simulink model "Reg_courant_RL_H26_2024"  (R2024a)
settings: Solver=ode4  StartTime=0.0  StopTime=inf  FixedStep=Ts  RelTol=1e-3
PostLoadFcn:
  | Reg_vitesse_courant_H24m;
InitFcn:
  | Reg_courant_RL_H26m;
values from neighbouring files (symbols this model uses):
  fperturbation = 1 / (2*pi*nc*Tel)    (= 200.494258843)    [Reg_courant_RL_H26m.m]
  Ian = 0.5    [Reg_courant_RL_H26m.m]
  Kamp = Gain_Ampli_Puissance(1)    [Reg_courant_RL_H26m.m]
  Kc = Gain_Capteur_Courant(1)    [Reg_courant_RL_H26m.m]
  Kel = 1 / Rel    (= 0.283808712927)    [Reg_courant_RL_H26m.m]
  limVampinf = -5    [Reg_courant_RL_H26m.m]
  limVampsup = 5    [Reg_courant_RL_H26m.m]
  PulseWidth = Tperturbcourant / 2    [Reg_courant_RL_H26m.m]
  Tech = Tel / nTechTel    [Reg_courant_RL_H26m.m]
  Tel = Lel / Rel    (= 7.93812970058e-05)    [Reg_courant_RL_H26m.m]
  Tperturbcourant = 4 * ceil(Ntau * Tel / Ts)    [Reg_courant_RL_H26m.m]
  Ts = Tel / nTsTel    (= 1.98453242515e-06)    [Reg_courant_RL_H26m.m]
libraries: simulink x4, slpidlib x2
settings Model: Creator=Philippe Viarouge  LastModifiedBy=guill
settings SolverCC: AlgebraicLoopSolver=TrustRegion
settings ModelReferenceCC: EnableRefExpFcnMdlSchedulingChecks=on
settings RTWCC: GPUComputeCapability=3.5  DLArmComputeVersion=19.05
settings ConfigComp: CovBoundaryAbsTol=1.0e-5

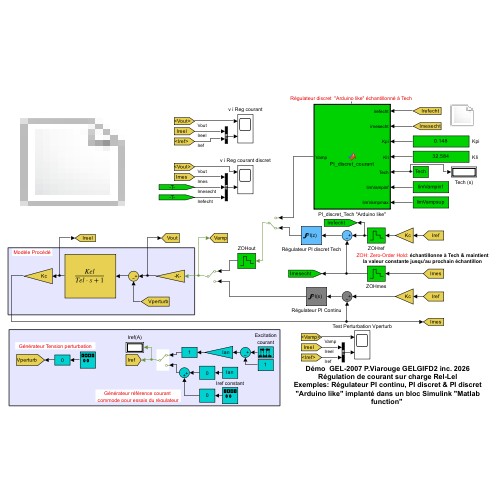
[thumbnail: Simulink's stored preview of the top-level diagram]
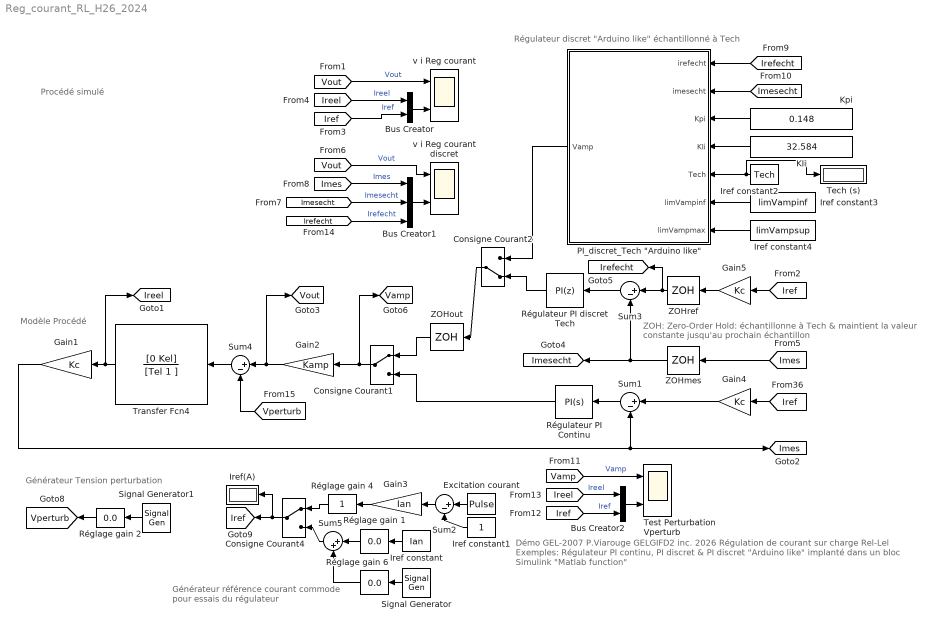
== system Reg_courant_RL_H26_2024 ==
  note: Modèle Procédé
  note: Générateur référence courant
      | commode pour essais du régulateur
  note: Générateur Tension perturbation
  note: Régulateur discret "Arduino like" échantillonné à Tech
  note: Procédé simulé
  note: Démo  GEL-2007 P.Viarouge GELGIFD2 inc. 2026
      | Régulation de courant sur charge Rel-Lel
      | Exemples: Régulateur PI continu, PI discret & PI discret "Arduino like" implanté dans un bloc Simulink "Matlab function"
  note: ZOH: Zero-Order Hold: échantillonne à Tech & maintient la valeur constante jusqu'au prochain échantillon
  " Consigne Courant1" : ManualSwitch
  " Consigne Courant2" : ManualSwitch  CurrentSetting=0
  " Consigne Courant4" : ManualSwitch
  Bus Creator : BusCreator  Inputs=2
  Bus Creator1 : BusCreator  Inputs=3
  Bus Creator2 : BusCreator  Inputs=2
  Excitation courant : DiscretePulseGenerator  Amplitude=2  Period=Tperturbcourant  PulseWidth=PulseWidth  PhaseDelay=PulseWidth  SampleTime=Ts
  Gain1 : Gain  Gain=Kc  SaturateOnIntegerOverflow=on  OutDataTypeStr=Inherit: Same as input  ParamDataTypeStr=Inherit: Same as input
  Gain2 : Gain  Gain=Kamp  SaturateOnIntegerOverflow=on  OutDataTypeStr=Inherit: Same as input  ParamDataTypeStr=Inherit: Same as input
  Gain3 : Gain  Gain=Ian  SaturateOnIntegerOverflow=on  OutDataTypeStr=Inherit: Same as input  ParamDataTypeStr=Inherit: Same as input
  Gain4 : Gain  Gain=Kc  SaturateOnIntegerOverflow=on  OutDataTypeStr=Inherit: Same as input  ParamDataTypeStr=Inherit: Same as input
  Gain5 : Gain  Gain=Kc  SaturateOnIntegerOverflow=on  OutDataTypeStr=Inherit: Same as input  ParamDataTypeStr=Inherit: Same as input
  Iref constant : Constant  Value=Ian
  Iref constant1 : Constant
  Iref constant2 : Constant  Value=Tech
  Iref constant3 : Constant  Value=limVampinf
  Iref constant4 : Constant  Value=limVampsup
  Iref(A) : Display
  KIi : Constant  Value=32.584
  Kpi : Constant  Value=0.148
  "PI_discret_Tech \"Arduino like\"" : MATLAB Function  TreatAsAtomicUnit=on
  Réglage gain 1 : simulink/Math Operations/Slider Gain  gain=0.0  low=0  high=1
  Réglage gain 2 : simulink/Math Operations/Slider Gain  gain=0.0  low=0  high=10
  Réglage gain 4 : simulink/Math Operations/Slider Gain  gain=1  low=0  high=2
  Réglage gain 6 : simulink/Math Operations/Slider Gain  gain=0.0  low=0  high=2
  Régulateur PI Continu : slpidlib/PID Controller  Controller=PI  Form=Parallel  TimeDomain=Continuous-time  UseExternalTs=off  SampleTime=Ts  IntegratorMethod=Forward Euler  FilterMethod=Forward Euler  ControllerParametersSource=internal  P=2.13202399414714  I=58536.4727696562  UseKiTs=off  D=-0.000553625934463325  UseExternalDerivativeSource=off  N=711.832973902977  UseFilter=on  TunerSelectOption=Transfer Function Based (PID Tuner App)  InitialConditionSource=internal  InitialConditionForIntegrator=0  InitialConditionForFilter=0  DifferentiatorICPrevScaledInput=0  ExternalReset=none  TrackingMode=off  Kt=1  LimitOutput=on  SatLimitsSource=internal  UpperSaturationLimit=limVampsup  LowerSaturationLimit=limVampinf  LinearizeAsGain=off  AntiWindupMode=clamping  Kb=1  LimitIntegrator=off  UpperIntegratorSaturationLimit=inf  LowerIntegratorSaturationLimit=-inf  POutMin=[]  POutMax=[]  IOutMin=[]  IOutMax=[]  DOutMin=[]  DOutMax=[]  NOutMin=[]  NOutMax=[]  SumOutMin=[]  SumOutMax=[]  SaturationOutDataTypeStr=Inherit: Inherit via back propagation  SaturationOutMin=[]  SaturationOutMax=[]  PParamMin=[]  PParamMax=[]  IParamMin=[]  IParamMax=[]  DParamMin=[]  DParamMax=[]  NParamMin=[]  NParamMax=[]  KbParamMin=[]  KbParamMax=[]  KtParamMin=[]  KtParamMax=[]  KbOutMin=[]  KbOutMax=[]  KtOutMin=[]  KtOutMax=[]  IntegratorOutMin=[]  IntegratorOutMax=[]  FilterOutMin=[]  FilterOutMax=[]  SumI1OutMin=[]  SumI1OutMax=[]  SumI2OutMin=[]  SumI2OutMax=[]  SumI3OutMin=[]  SumI3OutMax=[]  SumI4OutMin=[]  SumI4OutMax=[]  SumDOutMin=[]  SumDOutMax=[]  DifferentiatorOutMin=[]  DifferentiatorOutMax=[]  FilterDiffOutCoefMin=[]  FilterDiffOutCoefMax=[]  ReciprocalOutMin=[]  ReciprocalOutMax=[]  SumDenOutMin=[]  SumDenOutMax=[]  SumNumOutMin=[]  SumNumOutMax=[]  DivideOutMin=[]  DivideOutMax=[]  UdiffTsProdOutMin=[]  UdiffTsProdOutMax=[]  NTsProdOutMin=[]  NTsProdOutMax=[]  UintegralTsProdOutMin=[]  UintegralTsProdOutMax=[]  UngainTsProdOutMin=[]  UngainTsProdOutMax=[]  ClampingZeroOutDataTypeStr=Inherit: Inherit via back propagation  ClampingZeroOutMin=[]  ClampingZeroOutMax=[]  FilterDenConstantOutDataTypeStr=Inherit: Inherit via back propagation  FilterDenConstantOutMin=[]  FilterDenConstantOutMax=[]  PCopyOutDataTypeStr=Inherit: Inherit via back propagation  PCopyOutMin=[]  PCopyOutMax=[]  NCopyOutDataTypeStr=Inherit: Inherit via back propagation  NCopyOutMin=[]  NCopyOutMax=[]  IntegratorContinuousStateAttributes=''  IntegratorStateMustResolveToSignalObject=off  IntegratorRTWStateStorageClass=Auto  FilterContinuousStateAttributes=''  FilterStateMustResolveToSignalObject=off  FilterRTWStateStorageClass=Auto  ParallelPVariant=InternalParameters  IdealPVariant=Disabled  IVariant=InternalParameters  DVariant=Disabled  IntegratorVariant=Continuous  SatVariant=Enabled  AWVariant=ContClampingParallel  PCopyVariant=Disabled  TRVariant=Disabled  FdbkBlocksVariant=Forward  IdealPFdbkVariant=Disabled  SatFdbkVariant=Disabled  DerivativeFilterVariant=Disabled  NVariant=Disabled  NCopyVariant=Disabled_SignalSpec  FilterICVariant=Disabled  IntegratorICVariant=InternalICs  ExternalResetVariant=Disabled  TRSumVariant=Passthrough  SumFdbkVariant=Disabled  SumVariant=Sum_PI  TsampFilterVariant=InternalTs  TsampNgainVariant=Passthrough  TsampIntegralVariant=Disabled_SignalSpec  ExternalSaturationOutDataTypeStr=Inherit: Same as second input  DerivativeSourceVariant=Disabled
  Régulateur PI discret Tech : slpidlib/PID Controller  Controller=PI  Form=Parallel  TimeDomain=Discrete-time  UseExternalTs=off  SampleTime=Tech  IntegratorMethod=Forward Euler  FilterMethod=Forward Euler  ControllerParametersSource=internal  P=2.13202399414714  I=58536.4727696562  UseKiTs=off  D=-0.000553625934463325  UseExternalDerivativeSource=off  N=711.832973902977  UseFilter=on  TunerSelectOption=Transfer Function Based (PID Tuner App)  InitialConditionSource=internal  InitialConditionForIntegrator=0  InitialConditionForFilter=0  DifferentiatorICPrevScaledInput=0  ExternalReset=none  TrackingMode=off  Kt=1  LimitOutput=on  SatLimitsSource=internal  UpperSaturationLimit=limVampsup  LowerSaturationLimit=limVampinf  LinearizeAsGain=off  AntiWindupMode=clamping  Kb=1  LimitIntegrator=off  UpperIntegratorSaturationLimit=inf  LowerIntegratorSaturationLimit=-inf  POutMin=[]  POutMax=[]  IOutMin=[]  IOutMax=[]  DOutMin=[]  DOutMax=[]  NOutMin=[]  NOutMax=[]  SumOutMin=[]  SumOutMax=[]  SaturationOutDataTypeStr=Inherit: Inherit via back propagation  SaturationOutMin=[]  SaturationOutMax=[]  PParamMin=[]  PParamMax=[]  IParamMin=[]  IParamMax=[]  DParamMin=[]  DParamMax=[]  NParamMin=[]  NParamMax=[]  KbParamMin=[]  KbParamMax=[]  KtParamMin=[]  KtParamMax=[]  KbOutMin=[]  KbOutMax=[]  KtOutMin=[]  KtOutMax=[]  IntegratorOutMin=[]  IntegratorOutMax=[]  FilterOutMin=[]  FilterOutMax=[]  SumI1OutMin=[]  SumI1OutMax=[]  SumI2OutMin=[]  SumI2OutMax=[]  SumI3OutMin=[]  SumI3OutMax=[]  SumI4OutMin=[]  SumI4OutMax=[]  SumDOutMin=[]  SumDOutMax=[]  DifferentiatorOutMin=[]  DifferentiatorOutMax=[]  FilterDiffOutCoefMin=[]  FilterDiffOutCoefMax=[]  ReciprocalOutMin=[]  ReciprocalOutMax=[]  SumDenOutMin=[]  SumDenOutMax=[]  SumNumOutMin=[]  SumNumOutMax=[]  DivideOutMin=[]  DivideOutMax=[]  UdiffTsProdOutMin=[]  UdiffTsProdOutMax=[]  NTsProdOutMin=[]  NTsProdOutMax=[]  UintegralTsProdOutMin=[]  UintegralTsProdOutMax=[]  UngainTsProdOutMin=[]  UngainTsProdOutMax=[]  ClampingZeroOutDataTypeStr=Inherit: Inherit via back propagation  ClampingZeroOutMin=[]  ClampingZeroOutMax=[]  FilterDenConstantOutDataTypeStr=Inherit: Inherit via back propagation  FilterDenConstantOutMin=[]  FilterDenConstantOutMax=[]  PCopyOutDataTypeStr=Inherit: Inherit via back propagation  PCopyOutMin=[]  PCopyOutMax=[]  NCopyOutDataTypeStr=Inherit: Inherit via back propagation  NCopyOutMin=[]  NCopyOutMax=[]  IntegratorContinuousStateAttributes=''  IntegratorStateMustResolveToSignalObject=off  IntegratorRTWStateStorageClass=Auto  FilterContinuousStateAttributes=''  FilterStateMustResolveToSignalObject=off  FilterRTWStateStorageClass=Auto  ParallelPVariant=InternalParameters  IdealPVariant=Disabled  IVariant=InternalParameters  DVariant=Disabled  IntegratorVariant=Discrete  SatVariant=Enabled  AWVariant=DiscClampingParallel  PCopyVariant=Disabled  TRVariant=Disabled  FdbkBlocksVariant=Forward  IdealPFdbkVariant=Disabled  SatFdbkVariant=Disabled  DerivativeFilterVariant=Disabled  NVariant=Disabled  NCopyVariant=Disabled_SignalSpec  FilterICVariant=Disabled  IntegratorICVariant=InternalICs  ExternalResetVariant=Disabled  TRSumVariant=Passthrough  SumFdbkVariant=Disabled  SumVariant=Sum_PI  TsampFilterVariant=InternalTs  TsampNgainVariant=Passthrough  TsampIntegralVariant=Disabled_SignalSpec  ExternalSaturationOutDataTypeStr=Inherit: Same as second input  DerivativeSourceVariant=Disabled
  Signal Generator : SignalGenerator  Amplitude=Ian  Frequency=10
  Signal Generator1 : SignalGenerator  Frequency=fperturbation
  Sum{1..4} (4 alike) : Sum  Inputs=|+-
  Sum5 : Sum  Inputs=|++
  Tech (s) : Display
  Test Perturbation Vperturb : Scope  NumInputPorts=2
  Transfer Fcn4 : TransferFcn  Numerator=[0 Kel]  Denominator=[Tel 1 ]
  ZOHmes : ZeroOrderHold  SampleTime=Tech
  ZOHout : ZeroOrderHold  SampleTime=Tech
  ZOHref : ZeroOrderHold  SampleTime=Tech
  v i Reg courant : Scope  NumInputPorts=2
  v i Reg courant discret : Scope  NumInputPorts=2
  tag scope: Imes=global, Imesecht=global, Ireel=global, Iref=global, Irefecht=global, Vamp=global, Vout=global, Vperturb=global
  wires:
  Réglage gain 1/1 -> Sum5/1
  Sum5/1 -> " Consigne Courant4"/2
  Iref constant/1 -> Réglage gain 1/1
  Gain1/1 -> Sum1/2, [Imes]
  Réglage gain 4/1 -> " Consigne Courant4"/1
  Gain3/1 -> Réglage gain 4/1
  Gain4/1 -> Sum1/1
  Signal Generator/1 -> Réglage gain 6/1
  Transfer Fcn4/1 -> [Ireel], Gain1/1
  Réglage gain 6/1 -> Sum5/2
  [Iref] -> Gain4/1
  [Vout] -> v i Reg courant/1  "Vout"
  [Ireel] -> Bus Creator/1  "Ireel"
  [Iref] -> Bus Creator/2  "Iref"
  Bus Creator/1 -> v i Reg courant/2
  Excitation courant/1 -> Sum2/1
  Iref constant1/1 -> Sum2/2
  Sum2/1 -> Gain3/1
  Sum1/1 -> Régulateur PI Continu/1
  Régulateur PI Continu/1 -> " Consigne Courant1"/2
  Sum3/1 -> Régulateur PI discret Tech/1
  ZOHref/1 -> [Irefecht], Sum3/1
  ZOHmes/1 -> Sum3/2, [Imesecht]
  [Imes] -> ZOHmes/1
  ZOHout/1 -> " Consigne Courant1"/1
  Gain5/1 -> ZOHref/1
  [Iref] -> Gain5/1
  Bus Creator1/1 -> v i Reg courant discret/2
  [Imesecht] -> Bus Creator1/2  "Imesecht"
  [Vout] -> v i Reg courant discret/1  "Vout"
  [Imes] -> Bus Creator1/1  "Imes"
  [Irefecht] -> "PI_discret_Tech \"Arduino like\""/1(irefecht)
  [Imesecht] -> "PI_discret_Tech \"Arduino like\""/2(imesecht)
  "PI_discret_Tech \"Arduino like\""/1(Vamp) -> " Consigne Courant2"/1
  " Consigne Courant2"/1 -> ZOHout/1
  Régulateur PI discret Tech/1 -> " Consigne Courant2"/2
  Kpi/1 -> "PI_discret_Tech \"Arduino like\""/3(Kpi)
  KIi/1 -> "PI_discret_Tech \"Arduino like\""/4(KIi)
  Iref constant2/1 -> "PI_discret_Tech \"Arduino like\""/5(Tech), Tech (s)/1
  Iref constant3/1 -> "PI_discret_Tech \"Arduino like\""/6(limVampinf)
  Iref constant4/1 -> "PI_discret_Tech \"Arduino like\""/7(limVampmax)
  Sum4/1 -> Transfer Fcn4/1
  Gain2/1 -> [Vout], Sum4/1
  " Consigne Courant1"/1 -> Gain2/1, [Vamp]
  [Vamp] -> Test Perturbation Vperturb/1  "Vamp"
  Bus Creator2/1 -> Test Perturbation Vperturb/2
  [Iref] -> Bus Creator2/2  "Iref"
  [Ireel] -> Bus Creator2/1  "Ireel"
  [Irefecht] -> Bus Creator1/3  "Irefecht"
  Signal Generator1/1 -> Réglage gain 2/1
  Réglage gain 2/1 -> [Vperturb]
  [Vperturb] -> Sum4/2
  " Consigne Courant4"/1 -> Iref(A)/1, [Iref]

== matlab function Reg_courant_RL_H26_2024/PI_discret_Tech "Arduino like" ==
  data: irefecht input; Vamp output; imesecht input; Kpi input; KIi input; Tech input; limVampinf input; limVampmax input
function Vamp = PI_discret_courant(irefecht, imesecht, Kpi, KIi, Tech, limVampinf, limVampmax)
%P.Viarouge 06-03-26
% Régulateur PI discret à intégrateur explicite pour régulation de courant
%
% Remarque : les paramètres du régulateur (gains Kpi, KIi, période
% d'échantillonnage Tech, seuils des limiteurs de sortie du régulateur
% limVampinf et limVampmax) sont déclarés comme arguments de la fonction.
% Dans le bloc MATLAB Function de Simulink, ils apparaissent donc comme
% des entrées du bloc.
%
% Cela permet de relier ces entrées à des blocs Constant de Simulink,
% ce qui rend le réglage du régulateur simple et visible directement
% dans le schéma.
%
% Cette méthode est souvent plus pratique que de déclarer ces paramètres
% comme des variables internes ou des paramètres du bloc dans l’éditeur
% de la MATLAB Function, car elle permet d’ajuster les gains du régulateur
% directement depuis le modèle Simulink en changeant les valeurs de ces
% variables dans les blocs Constant "à la volée" pendant la simulation
% en mode permanent (avec StopTime = tinf).
%
% ENTREES :
%   irefecht   : courant de référence échantillonné (ZOH à Tech)
%   imesecht   : courant mesuré échantillonné (ZOH à Tech)
%   Kpi        : gain proportionnel du PI
%   KIi        : gain intégral du PI
%   Tech       : période d'échantillonnage
%   limVampinf : limite basse de la commande : limiteur de sortie du PI
%   limVampmax : limite haute de la commande : limiteur de sortie du PI
%
% SORTIE :
%   Vamp       : signal de commande amplificateur de gain Kamp
%
% EQUATIONS DISCRETES DU PI IMPLANTEES :
%   e(k)        = irefecht(k) - imesecht(k)     % erreur de courant
%   xI(k)       = xI(k-1) + Tech*e(k)           % état intégrateur discret
%   Vamp_ns(k)  = Kpi*e(k) + KIi*xI(k)          % commande non saturée
%   Vamp(k)     = saturation( Vamp_ns(k) )      % commande réellement appliquée
%
% Ici, l'intégrateur est explicite : la variable xI représente directement
% l'intégrale discrète de l'erreur. Cela rend l'interprétation physique
% et la gestion de l'anti-windup plus claires
%
% Variables persistantes = mémoire du régulateur entre deux échantillons
% prélevés à Tech. Variables déclarées persistent dans la fonction.
% Signification : elles conservent leur valeur entre deux appels
% de la fonction.
%
% xIi    : état intégrateur discret du régulateur
% eiprec : erreur précédente (utile ici surtout pour mémoire/observation,
%          même si la formulation PI explicite de l'intégrateur 
%          n'en a pas nécessairement besoin)
persistent xIi eiprec

% Initialisation xIi et eiprec au début de la simulation
% Au premier appel de la fonction, ces variables persistent n’existent pas
% encore. Elles sont donc vides. La fonction isempty() permet de détecter
% cette situation.
if isempty(xIi)
    xIi = 0;
end
if isempty(eiprec)
    eiprec = 0;
end

% Calcul de l'erreur de courant pour l'échantillon courant
ei = irefecht - imesecht;

% -------------------------------------------------------------------------
% CALCUL PROVISOIRE DE L'ETAT INTEGRATEUR
% On calcule d'abord la valeur "candidate" de l'intégrateur à l'instant k :
% xIi_new = xIi(k-1) + Tech*e(k)
%
% Cette valeur n'est pas encore validée définitivement car on doit d'abord
% vérifier si elle conduit à une commande non saturée qui aggrave
% une saturation déjà présente.
% -------------------------------------------------------------------------
xIi_new = xIi + Tech*ei;

% Calcul de la commande "non saturée" (la saturation est appliquée après)
% Vamp_ns : commande calculée par le PI avant limitation
Vamp_ns = Kpi*ei + KIi*xIi_new;

% Application du limiteur après détection de la saturation de la commande
if Vamp_ns > limVampmax
    Vamp = limVampmax;
elseif Vamp_ns < limVampinf
    Vamp = limVampinf;
else
    Vamp = Vamp_ns;
end

% -------------------------------------------------------------------------
% GESTION DE L'ANTI-WINDUP DU REGULATEUR
%
% Si la commande non saturée Vamp_ns dépasse la limite haute et que l'erreur
% ei est positive, cela signifie que le régulateur voudrait encore
% augmenter la commande alors que la sortie réelle est déjà bloquée
% au maximum.
%
% De même, si Vamp_ns est inférieure à la limite basse et que l'erreur ei
% est négative, le régulateur voudrait encore diminuer la commande alors
% que la sortie réelle est déjà bloquée au minimum.
%
% Dans ces deux cas, on n'actualise pas l'état intégrateur xIi.
% On évite ainsi que l'intégrale de l'erreur continue à s'accumuler
% dans le sens qui aggrave la saturation.
%
% C'est le phénomène classique de "windup" : quand l’erreur disparaît
% ou change de signe, le régulateur a accumulé trop d’action intégrale
% et met longtemps à revenir à un fonctionnement normal.
%
% En revanche, si l'erreur tend à faire revenir la commande vers la zone
% non saturée, on autorise la mise à jour normale de l'intégrateur.
% -------------------------------------------------------------------------
if (Vamp_ns > limVampmax && ei > 0) || (Vamp_ns < limVampinf && ei < 0)
    % La commande calculée avant saturation dépasse une limite et
    % l'erreur pousse encore dans cette même direction.
    % Cela aggraverait la saturation : on fige donc l'intégrateur
    % (on ne met pas à jour xIi).
else
    % Situation normale : la commande n'aggrave pas la saturation
    % (ou bien l'erreur aide à en sortir).
    % On valide alors la nouvelle valeur de l'intégrateur.
    xIi = xIi_new;
end

% Mise à jour de l'erreur précédente pour le prochain échantillon
eiprec = ei;

% -------------------------------------------------------------------------
% REMARQUE IMPORTANTE
% TRANSPOSITION DE CE CODE DANS LE CODE DU REGULATEUR PI DANS L'ARDUINO
%
% La structure de ce régulateur PI discret est directement transposable
% dans un microcontrôleur comme l'Arduino. Dans l’Arduino, l’équivalent
% pratique du fonctionnement discret simulé avec le ZOH et le PID discret
% est un timer matériel qui déclenche une ISR à période constante
% (consulter la documentation Arduino).
%
% TOUT CODE de PID discret BASÉ sur loop() OU delay() DOIT ETRE PROSCRIT,
% car il ne garantit pas une période d’échantillonnage constante Tech.
% UN RÉGULATUR DISCRET SUR ARDUINO DOIT ÊTRE EXÉCUTÈ PÉRIODIQUEMENT à Tech
% cCONSTANTE par un TIMER  via une INTERRUTION (ISR).
%
% Le code de cette fonction correspond exactement à l'algorithme exécuté
% à chaque période d'échantillonnage Tech :
%   1) lecture du capteur (courant mesuré)
%   2) calcul de l'erreur
%   3) mise à jour de l'intégrateur discret
%   4) calcul de la commande PI discrète
%   5) application de la saturation
%   6) mémorisation des variables pour l'échantillon suivant
%
% Les variables "persistent" jouent le rôle de mémoire du régulateur
% entre deux instants d'échantillonnage.
%
% Dans une implantation Arduino, ce calcul est exécuté périodiquement
% toutes les Tech secondes (par exemple dans une interruption timer gérée
% avec ISR), ce qui reproduit exactement le comportement simulé dans
% Simulink (et vice-versa).
% -------------------------------------------------------------------------
